simulink model "ovap_sim"  (R2025a)
settings: Solver=ode4  StartTime=0.0  StopTime=20  FixedStep=0.002  RelTol=1e-3
undefined symbols (not defined in the file): X, Y, Z
libraries: sm_lib x173, nesl_utility x72, simulink_extras x37, slpidlib x16, fl_lib x2
(part 1 of 5)
settings Model: Creator=Khang  LastModifiedBy=Khang
settings ExplorerConfigSet: InternalSimMechanicsExplorerSettings=|
  | <ExplorerConfiguration>
  | 
  |   <canonicalview>aerospace</canonicalview>
  | 
  |   <TilePanel>
  |     <TileInfo>
  |       <Tiles Columns="1" Count="1" Height="660" Rows="1" Width="1083">
  |         <Row Weight="1"/>
  |         <Column Weight="1"/>
  |         <Tile Height="1" Width="1" X="0" Y="0"/>
  |       </Tiles>
  |     </TileInfo>
  |     <SceneInfo>
  |       <SceneViewer>
  |         <IsThisViewStd>
  |           <IsStandardView>off</IsStandardView>
  |           <StandardViewName>Front</StandardViewName>
  |         </IsThisViewStd>
  |         <BGColor>
  |           <R>1</R>
  |           <G>1</G>
  |           <B>1</B>
  |           <A>1</A>
  |         </BGColor>
  |         <Camera>
  |           <DoPerspective>off</DoPerspective>
  |           <Position>
  |             <X>1.8079000547306572</X>
  |             <Y>1.5417221131491254</Y>
  |             <Z>-1.2061321654562736</Z>
  |           </Position>
  |           <Center>
  |             <X>0.0050000039551827725</X>
  |             <Y>-0.00041913422088184807</Y>
  |             <Z>-4.5055192872524335e-09</Z>
  |           </Center>
  |           <Up>
  |             <X>-0.32558894990861931</X>
  |             <Y>-0.31626154677303076</Y>
  |             <Z>-0.891050206065928</Z>
  |           </Up>
  |           <XLim>0.25728389340937141</XLim>
  |           <YLim>0.25728389340937141</YLim>
  |           <ViewLimDist>0.01</ViewLimDist>
  |         </Camera>
  |       </SceneViewer>
  |     </SceneInfo>
  |   </TilePanel>
  | 
  |   <MechEditorPanel>
  |     <GfxPanelCameraMap/>
  |     <Cameras/>
  |     <VideoCreator>
  |       <IncludeTiles>All</IncludeTiles>
  |       <IncludeTime>on</IncludeTime>
  |       <IncludeWorldFrame>off</IncludeWorldFrame>
  |       <PlaybackSpeedRatio>1</PlaybackSpeedRatio>
  |       <FrameRate>30</FrameRate>
  |       <FrameSize>auto</FrameSize>
  |       <VideoFormat>UncompressedAVI</VideoFormat>
  |     </VideoCreator>
  |   </MechEditorPanel>
  | 
  |   <PlaybackSettings>
  |     <PlaybackSpeedFactor>1</PlaybackSpeedFactor>
  |   </PlaybackSettings>
  | 
  | </ExplorerConfiguration>

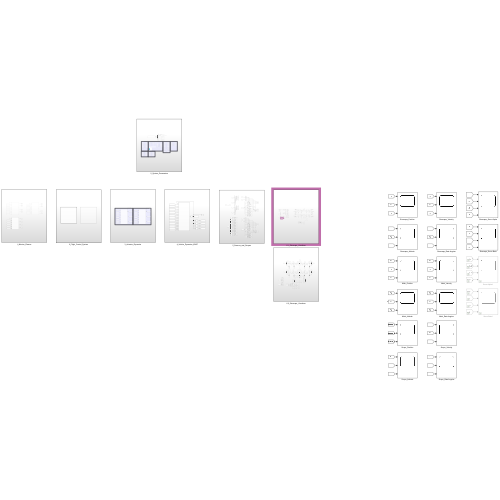
[thumbnail: Simulink's stored preview of the top-level diagram]
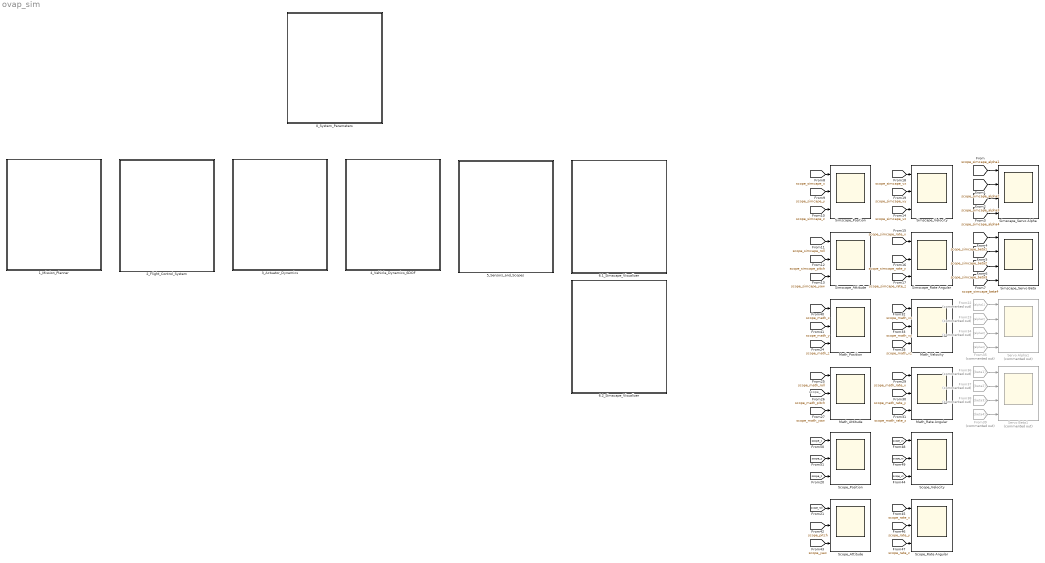
== system ovap_sim ==
  note: scope_
  0_System_Parameters : Subsystem
  1_Mission_Planner : Subsystem
  2_Flight_Control_System : Subsystem
  3_Actuator_Dynamics : Subsystem
  4_Vehicle_Dynamics_6DOF : Subsystem
  5_Sensors_and_Scopes : Subsystem
  6.1_Simscape_Visualizer : Subsystem
  6.2_Simscape_Visualizer : Subsystem
  From22 : From  Commented=on  GotoTag=alpha1
  From23 : From  Commented=on  GotoTag=alpha2
  From34 : From  Commented=on  GotoTag=alpha3
  From35 : From  Commented=on  GotoTag=alpha4
  From36 : From  Commented=on  GotoTag=beta1
  From37 : From  Commented=on  GotoTag=beta2
  From38 : From  Commented=on  GotoTag=beta3
  From39 : From  Commented=on  GotoTag=beta4
  Math_Attitude : Scope  NumInputPorts=3
      settings: ActiveDisplayYMinimum=-221.23870435466742  ActiveDisplayYMaximum=1941.5029004107885  DataLoggingVariableName=ScopeData32
  Math_Position : Scope  NumInputPorts=3
      settings: ActiveDisplayYMinimum=-1  ActiveDisplayYMaximum=1  DataLoggingVariableName=ScopeData34
  Math_Rate Angular : Scope  NumInputPorts=3
      settings: ActiveDisplayYMinimum=-1.0728968264760348E-15  ActiveDisplayYMaximum=6.562124395111157E-16  DataLoggingVariableName=ScopeData35
  Math_Velocity : Scope  NumInputPorts=3
      settings: ActiveDisplayYMinimum=-2.0436694374784938  ActiveDisplayYMaximum=7.1181854930531765  DataLoggingVariableName=ScopeData38
  Scope_Attitude : Scope  NumInputPorts=3
      settings: ActiveDisplayString=3  ActiveDisplayYMinimum=-2.4868538922904428  ActiveDisplayYMaximum=22.252327579018413  DataLoggingVariableName=ScopeData16
  Scope_Position : Scope  NumInputPorts=3
      settings: ActiveDisplayString=3  ActiveDisplayYMinimum=-1.3579834876063737  ActiveDisplayYMaximum=11.844828712328191  DataLoggingVariableName=ScopeData4
  Scope_Rate Angular : Scope  NumInputPorts=3
      settings: ActiveDisplayString=3  ActiveDisplayYMinimum=-0.388418902791342  ActiveDisplayYMaximum=0.27906120373033161  DataLoggingVariableName=ScopeData17
  Scope_Velocity : Scope  NumInputPorts=3
      settings: ActiveDisplayString=3  ActiveDisplayYMinimum=-3.4139647268091498  ActiveDisplayYMaximum=3.4772220698527239  DataLoggingVariableName=ScopeData2
  Servo Alpha1 : Scope  Commented=on  NumInputPorts=4
      settings: ActiveDisplayYMinimum=-3.9267300095298534  ActiveDisplayYMaximum=3.9256735239341554  DataLoggingVariableName=ScopeData36
  Servo Beta1 : Scope  Commented=on  NumInputPorts=4
      settings: ActiveDisplayYMinimum=-3.9267300095298534  ActiveDisplayYMaximum=3.9256735239341554  DataLoggingVariableName=ScopeData37
  Simscape_Attitude : Scope  NumInputPorts=3
      settings: ActiveDisplayYMinimum=-10.100227257036986  ActiveDisplayYMaximum=78.44868955498238
  Simscape_Position : Scope  NumInputPorts=3
      settings: ActiveDisplayYMinimum=-8.4800718375241177E-15  ActiveDisplayYMaximum=3.4315544615870859E-14
  Simscape_Rate Angular : Scope  NumInputPorts=3
      settings: ActiveDisplayYMinimum=-143.23944878270581  ActiveDisplayYMaximum=143.23944878270581  DataLoggingVariableName=ScopeData3
  Simscape_Servo Alpha : Scope  NumInputPorts=4
      settings: ActiveDisplayYMinimum=-3.9267300095298534  ActiveDisplayYMaximum=3.9256735239341554  DataLoggingVariableName=ScopeData5
  Simscape_Servo Beta : Scope  NumInputPorts=4
      settings: ActiveDisplayYMinimum=-3.9267300095298534  ActiveDisplayYMaximum=3.9256735239341554  DataLoggingVariableName=ScopeData6
  Simscape_Velocity : Scope  NumInputPorts=3
      settings: ActiveDisplayYMinimum=-143.23944878270581  ActiveDisplayYMaximum=143.23944878270581  DataLoggingVariableName=ScopeData7
  wires:
  [scope_simcape_alpha1] -> Simscape_Servo Alpha/1
  [scope_simcape_alpha2] -> Simscape_Servo Alpha/2
  [scope_simcape_alpha3] -> Simscape_Servo Alpha/3
  [scope_simcape_alpha4] -> Simscape_Servo Alpha/4
  [scope_simcape_beta1] -> Simscape_Servo Beta/1
  [scope_simcape_beta2] -> Simscape_Servo Beta/2
  [scope_simcape_beta3] -> Simscape_Servo Beta/3
  [scope_simcape_beta4] -> Simscape_Servo Beta/4
  [scope_simcape_x] -> Simscape_Position/1
  [scope_simcape_y] -> Simscape_Position/2
  [scope_simcape_z] -> Simscape_Position/3
  [scope_simcape_roll] -> Simscape_Attitude/1
  [scope_simcape_pitch] -> Simscape_Attitude/2
  [scope_simcape_yaw] -> Simscape_Attitude/3
  [scope_simcape_rate_y] -> Simscape_Rate Angular/2
  [scope_simcape_rate_z] -> Simscape_Rate Angular/3
  [scope_simcape_vy] -> Simscape_Velocity/2
  [scope_simcape_vx] -> Simscape_Velocity/1
  [scope_simcape_vz] -> Simscape_Velocity/3
  [scope_simcape_rate_x] -> Simscape_Rate Angular/1
  [scope_math_vy] -> Math_Velocity/2
  From37/1 -> Servo Beta1/2
  From34/1 -> Servo Alpha1/3
  [scope_math_y] -> Math_Position/2
  From36/1 -> Servo Beta1/1
  From22/1 -> Servo Alpha1/1
  [scope_math_pitch] -> Math_Attitude/2
  [scope_math_rate_y] -> Math_Rate Angular/2
  From38/1 -> Servo Beta1/3
  [scope_math_x] -> Math_Position/1
  [scope_math_vx] -> Math_Velocity/1
  [scope_math_roll] -> Math_Attitude/1
  [scope_math_rate_z] -> Math_Rate Angular/3
  [scope_math_vz] -> Math_Velocity/3
  From35/1 -> Servo Alpha1/4
  [scope_math_yaw] -> Math_Attitude/3
  From23/1 -> Servo Alpha1/2
  [scope_math_z] -> Math_Position/3
  [scope_math_rate_x] -> Math_Rate Angular/1
  From39/1 -> Servo Beta1/4
  [scope_rate_y] -> Scope_Rate Angular/2
  [scope_rate_z] -> Scope_Rate Angular/3
  [scope_rate_x] -> Scope_Rate Angular/1
  [scope_vy] -> Scope_Velocity/2
  [scope_yaw] -> Scope_Attitude/3
  [scope_roll] -> Scope_Attitude/1
  [scope_vz] -> Scope_Velocity/3
  [scope_vx] -> Scope_Velocity/1
  [scope_z] -> Scope_Position/3
  [scope_x] -> Scope_Position/1
  [scope_pitch] -> Scope_Attitude/2
  [scope_y] -> Scope_Position/2

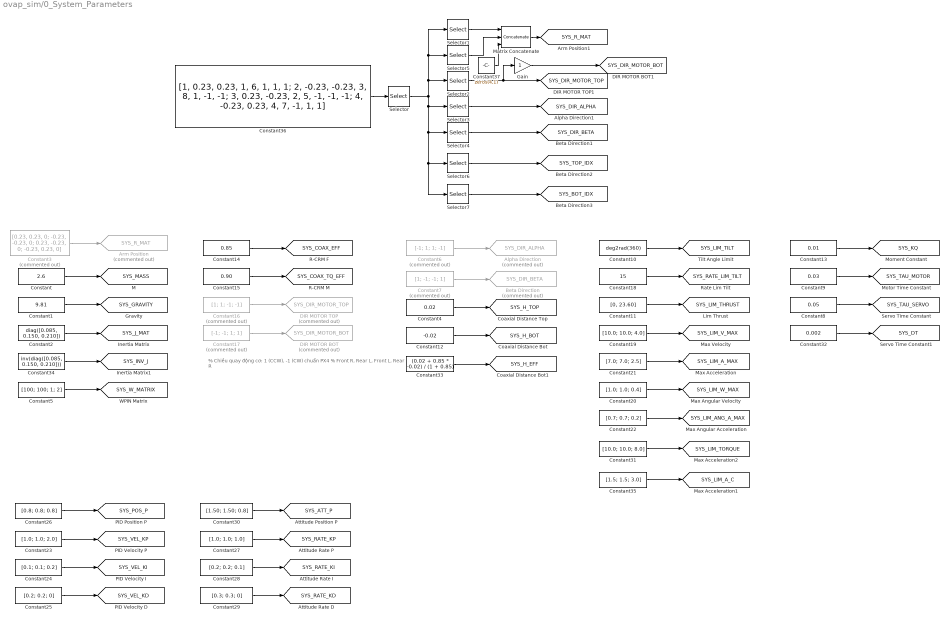
== system ovap_sim/0_System_Parameters ==
  note: % Chiều quay động cơ: 1 (CCW), -1 (CW) chuẩn PX4
      | % Front R, Rear L, Front L, Rear R
  Alpha Direction : Goto  Commented=on  GotoTag=SYS_DIR_ALPHA  TagVisibility=global
  Arm Position : Goto  Commented=on  GotoTag=SYS_R_MAT  TagVisibility=global
  Beta Direction : Goto  Commented=on  GotoTag=SYS_DIR_BETA  TagVisibility=global
  Constant : Constant  Value=2.6
  Constant1 : Constant  Value=9.81
  Constant10 : Constant  Value=deg2rad(360)
  Constant11 : Constant  Value=[0, 23.60]
  Constant12 : Constant  Value=-0.02
  Constant13 : Constant  Value=0.01
  Constant14 : Constant  Value=0.85
  Constant15 : Constant  Value=0.90
  Constant16 : Constant  Commented=on  Value=[1; 1; -1; -1]
  Constant17 : Constant  Commented=on  Value=[-1; -1; 1; 1]
  Constant18 : Constant  Value=15
  Constant19 : Constant  Value=[10.0; 10.0; 4.0]
  Constant2 : Constant  Value=diag([0.085, 0.150, 0.210])
  Constant20 : Constant  Value=[1.0; 1.0; 0.4]
  Constant21 : Constant  Value=[7.0; 7.0; 2.5]
  Constant22 : Constant  Value=[0.7; 0.7; 0.2]
  Constant23 : Constant  Value=[1.0; 1.0; 2.0]
  Constant24 : Constant  Value=[0.1; 0.1; 0.2]
  Constant25 : Constant  Value=[0.2; 0.2; 0]
  Constant26 : Constant  Value=[0.8; 0.8; 0.8]
  Constant27 : Constant  Value=[1.0; 1.0; 1.0]
  Constant28 : Constant  Value=[0.2; 0.2; 0.1]
  Constant29 : Constant  Value=[0.3; 0.3; 0]
  Constant3 : Constant  Commented=on  Value=[0.23, 0.23, 0; -0.23, -0.23, 0; 0.23, -0.23, 0; -0.23, 0.23, 0]
  Constant30 : Constant  Value=[1.50; 1.50; 0.8]
  Constant31 : Constant  Value=[10.0; 10.0; 8.0]
  Constant32 : Constant  Value=0.002
  Constant33 : Constant  Value=(0.02 + 0.85 * -0.02) / (1 + 0.85)
  Constant34 : Constant  Value=inv(diag([0.085, 0.150, 0.210]))
  Constant35 : Constant  Value=[1.5; 1.5; 3.0]
  Constant36 : Constant  Value=|
      | [1,  0.23,  0.23, 1, 6,  1,  1,  1; 
      |  2, -0.23, -0.23, 3, 8,  1, -1, -1; 
      |  3,  0.23, -0.23, 2, 5, -1, -1, -1; 
      |  4, -0.23,  0.23, 4, 7, -1,  1,  1]
  Constant37 : Constant  Value=zeros(4,1)
  Constant4 : Constant  Value=0.02
  Constant5 : Constant  Value=[100; 100; 1; 2]
  Constant6 : Constant  Commented=on  Value=[-1; 1; 1; -1]
  Constant7 : Constant  Commented=on  Value=[1; -1; -1; 1]
  Constant8 : Constant  Value=0.05
  Constant9 : Constant  Value=0.03
  DIR MOTOR BOT : Goto  Commented=on  GotoTag=SYS_DIR_MOTOR_BOT  TagVisibility=global
  DIR MOTOR TOP : Goto  Commented=on  GotoTag=SYS_DIR_MOTOR_TOP  TagVisibility=global
  Gain : Gain
  Matrix Concatenate : Concatenate  NumInputs=3  Mode=Multidimensional array  ConcatenateDimension=2
  Selector : Selector  NumberOfDimensions=2  InputPortWidth=3  IndexOptions=Select all,Index vector (dialog)  Indices=[1 3],[2 3 4 5 6 7 8]  OutputSizes=1,1
  Selector1 : Selector  NumberOfDimensions=2  InputPortWidth=3  IndexOptions=Select all,Index vector (dialog)  Indices=[1 3],1  OutputSizes=1,1
  Selector2 : Selector  NumberOfDimensions=2  InputPortWidth=3  IndexOptions=Select all,Index vector (dialog)  Indices=[1 3],5  OutputSizes=1,1
  Selector3 : Selector  NumberOfDimensions=2  InputPortWidth=3  IndexOptions=Select all,Index vector (dialog)  Indices=[1 3],6  OutputSizes=1,1
  Selector4 : Selector  NumberOfDimensions=2  InputPortWidth=3  IndexOptions=Select all,Index vector (dialog)  Indices=[1 3],7  OutputSizes=1,1
  Selector5 : Selector  NumberOfDimensions=2  InputPortWidth=3  IndexOptions=Select all,Index vector (dialog)  Indices=[1 3],2  OutputSizes=1,1
  Selector6 : Selector  NumberOfDimensions=2  InputPortWidth=3  IndexOptions=Select all,Index vector (dialog)  Indices=[1 3],3  OutputSizes=1,1
  Selector7 : Selector  NumberOfDimensions=2  InputPortWidth=3  IndexOptions=Select all,Index vector (dialog)  Indices=[1 3],4  OutputSizes=1,1
  tag scope: SYS_ATT_P=global, SYS_BOT_IDX=global, SYS_COAX_EFF=global, SYS_COAX_TQ_EFF=global, SYS_DIR_ALPHA=global, SYS_DIR_BETA=global, SYS_DIR_MOTOR_BOT=global, SYS_DIR_MOTOR_TOP=global, SYS_DT=global, SYS_GRAVITY=global, SYS_H_BOT=global, SYS_H_EFF=global, SYS_H_TOP=global, SYS_INV_J=global, SYS_J_MAT=global, SYS_KQ=global, SYS_LIM_ANG_A_MAX=global, SYS_LIM_A_C=global, SYS_LIM_A_MAX=global, SYS_LIM_THRUST=global, SYS_LIM_TILT=global, SYS_LIM_TORQUE=global, SYS_LIM_V_MAX=global, SYS_LIM_W_MAX=global, SYS_MASS=global, SYS_POS_P=global, SYS_RATE_KD=global, SYS_RATE_KI=global, SYS_RATE_KP=global, SYS_RATE_LIM_TILT=global, SYS_R_MAT=global, SYS_TAU_MOTOR=global, SYS_TAU_SERVO=global, SYS_TOP_IDX=global, SYS_VEL_KD=global, SYS_VEL_KI=global, SYS_VEL_KP=global, SYS_W_MATRIX=global
  wires:
  Constant/1 -> [SYS_MASS]
  Constant1/1 -> [SYS_GRAVITY]
  Constant2/1 -> [SYS_J_MAT]
  Constant3/1 -> Arm Position/1
  Constant5/1 -> [SYS_W_MATRIX]
  Constant6/1 -> Alpha Direction/1
  Constant7/1 -> Beta Direction/1
  Constant9/1 -> [SYS_TAU_MOTOR]
  Constant8/1 -> [SYS_TAU_SERVO]
  Constant10/1 -> [SYS_LIM_TILT]
  Constant11/1 -> [SYS_LIM_THRUST]
  Constant4/1 -> [SYS_H_TOP]
  Constant12/1 -> [SYS_H_BOT]
  Constant13/1 -> [SYS_KQ]
  Constant14/1 -> [SYS_COAX_EFF]
  Constant15/1 -> [SYS_COAX_TQ_EFF]
  Constant17/1 -> DIR MOTOR BOT/1
  Constant16/1 -> DIR MOTOR TOP/1
  Constant18/1 -> [SYS_RATE_LIM_TILT]
  Constant21/1 -> [SYS_LIM_A_MAX]
  Constant20/1 -> [SYS_LIM_W_MAX]
  Constant19/1 -> [SYS_LIM_V_MAX]
  Constant22/1 -> [SYS_LIM_ANG_A_MAX]
  Constant23/1 -> [SYS_VEL_KP]
  Constant24/1 -> [SYS_VEL_KI]
  Constant26/1 -> [SYS_POS_P]
  Constant25/1 -> [SYS_VEL_KD]
  Constant28/1 -> [SYS_RATE_KI]
  Constant29/1 -> [SYS_RATE_KD]
  Constant30/1 -> [SYS_ATT_P]
  Constant27/1 -> [SYS_RATE_KP]
  Constant31/1 -> [SYS_LIM_TORQUE]
  Constant32/1 -> [SYS_DT]
  Constant33/1 -> [SYS_H_EFF]
  Constant34/1 -> [SYS_INV_J]
  Constant35/1 -> [SYS_LIM_A_C]
  Constant36/1 -> Selector/1
  Selector/1 -> Selector7/1, Selector6/1, Selector4/1, Selector3/1, Selector2/1, Selector1/1, Selector5/1
  Selector2/1 -> Gain/1, [SYS_DIR_MOTOR_TOP]
  Selector3/1 -> [SYS_DIR_ALPHA]
  Selector4/1 -> [SYS_DIR_BETA]
  Constant37/1 -> Matrix Concatenate/3
  Selector1/1 -> Matrix Concatenate/1
  Matrix Concatenate/1 -> [SYS_R_MAT]
  Selector5/1 -> Matrix Concatenate/2
  Selector6/1 -> [SYS_TOP_IDX]
  Selector7/1 -> [SYS_BOT_IDX]
  Gain/1 -> [SYS_DIR_MOTOR_BOT]

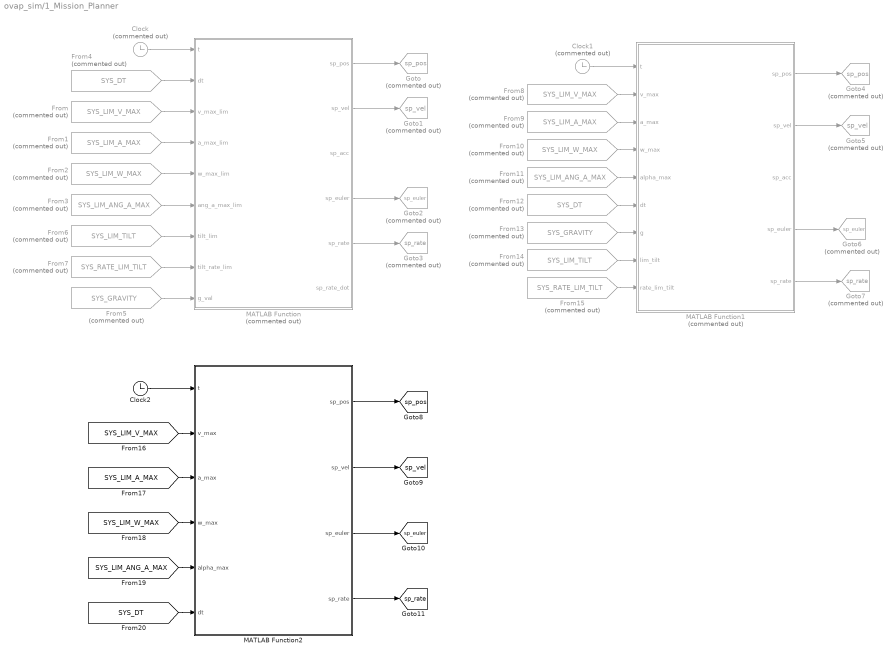
== system ovap_sim/1_Mission_Planner ==
  Clock : Clock  Commented=on
  Clock1 : Clock  Commented=on
  Clock2 : Clock
  From : From  Commented=on  GotoTag=SYS_LIM_V_MAX  TagVisibility=global
  From1 : From  Commented=on  GotoTag=SYS_LIM_A_MAX  TagVisibility=global
  From10 : From  Commented=on  GotoTag=SYS_LIM_W_MAX  TagVisibility=global
  From11 : From  Commented=on  GotoTag=SYS_LIM_ANG_A_MAX  TagVisibility=global
  From12 : From  Commented=on  GotoTag=SYS_DT  TagVisibility=global
  From13 : From  Commented=on  GotoTag=SYS_GRAVITY  TagVisibility=global
  From14 : From  Commented=on  GotoTag=SYS_LIM_TILT  TagVisibility=global
  From15 : From  Commented=on  GotoTag=SYS_RATE_LIM_TILT  TagVisibility=global
  From2 : From  Commented=on  GotoTag=SYS_LIM_W_MAX  TagVisibility=global
  From3 : From  Commented=on  GotoTag=SYS_LIM_ANG_A_MAX  TagVisibility=global
  From4 : From  Commented=on  GotoTag=SYS_DT  TagVisibility=global
  From5 : From  Commented=on  GotoTag=SYS_GRAVITY  TagVisibility=global
  From6 : From  Commented=on  GotoTag=SYS_LIM_TILT  TagVisibility=global
  From7 : From  Commented=on  GotoTag=SYS_RATE_LIM_TILT  TagVisibility=global
  From8 : From  Commented=on  GotoTag=SYS_LIM_V_MAX  TagVisibility=global
  From9 : From  Commented=on  GotoTag=SYS_LIM_A_MAX  TagVisibility=global
  Goto : Goto  Commented=on  GotoTag=sp_pos  TagVisibility=global
  Goto1 : Goto  Commented=on  GotoTag=sp_vel  TagVisibility=global
  Goto2 : Goto  Commented=on  GotoTag=sp_euler  TagVisibility=global
  Goto3 : Goto  Commented=on  GotoTag=sp_rate  TagVisibility=global
  Goto4 : Goto  Commented=on  GotoTag=sp_pos  TagVisibility=global
  Goto5 : Goto  Commented=on  GotoTag=sp_vel  TagVisibility=global
  Goto6 : Goto  Commented=on  GotoTag=sp_euler  TagVisibility=global
  Goto7 : Goto  Commented=on  GotoTag=sp_rate  TagVisibility=global
  MATLAB Function : MATLAB Function  Commented=on  TreatAsAtomicUnit=on
  MATLAB Function1 : MATLAB Function  Commented=on  TreatAsAtomicUnit=on
  MATLAB Function2 : MATLAB Function  TreatAsAtomicUnit=on
  tag scope: sp_euler=global, sp_pos=global, sp_rate=global, sp_vel=global
  wires:
  MATLAB Function/1(sp_pos) -> Goto/1
  MATLAB Function/5(sp_rate) -> Goto3/1
  MATLAB Function/2(sp_vel) -> Goto1/1
  MATLAB Function/4(sp_euler) -> Goto2/1
  From15/1 -> MATLAB Function1/9(rate_lim_tilt)
  From11/1 -> MATLAB Function1/5(alpha_max)
  From13/1 -> MATLAB Function1/7(g)
  MATLAB Function1/5(sp_rate) -> Goto7/1
  From9/1 -> MATLAB Function1/3(a_max)
  From12/1 -> MATLAB Function1/6(dt)
  From14/1 -> MATLAB Function1/8(lim_tilt)
  Clock1/1 -> MATLAB Function1/1(t)
  MATLAB Function1/2(sp_vel) -> Goto5/1
  From10/1 -> MATLAB Function1/4(w_max)
  MATLAB Function1/1(sp_pos) -> Goto4/1
  MATLAB Function1/4(sp_euler) -> Goto6/1
  From8/1 -> MATLAB Function1/2(v_max)
  Clock/1 -> MATLAB Function/1(t)
  From4/1 -> MATLAB Function/2(dt)
  From/1 -> MATLAB Function/3(v_max_lim)
  From1/1 -> MATLAB Function/4(a_max_lim)
  From2/1 -> MATLAB Function/5(w_max_lim)
  From3/1 -> MATLAB Function/6(ang_a_max_lim)
  From6/1 -> MATLAB Function/7(tilt_lim)
  From7/1 -> MATLAB Function/8(tilt_rate_lim)
  From5/1 -> MATLAB Function/9(g_val)
  MATLAB Function2/3(sp_euler) -> [sp_euler]
  [SYS_LIM_W_MAX] -> MATLAB Function2/4(w_max)
  [SYS_DT] -> MATLAB Function2/6(dt)
  Clock2/1 -> MATLAB Function2/1(t)
  [SYS_LIM_V_MAX] -> MATLAB Function2/2(v_max)
  [SYS_LIM_A_MAX] -> MATLAB Function2/3(a_max)
  [SYS_LIM_ANG_A_MAX] -> MATLAB Function2/5(alpha_max)
  MATLAB Function2/2(sp_vel) -> [sp_vel]
  MATLAB Function2/4(sp_rate) -> [sp_rate]
  MATLAB Function2/1(sp_pos) -> [sp_pos]

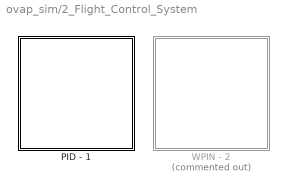
== system ovap_sim/2_Flight_Control_System ==
  PID - 1 : Subsystem
  WPIN - 2 : Subsystem  Commented=on

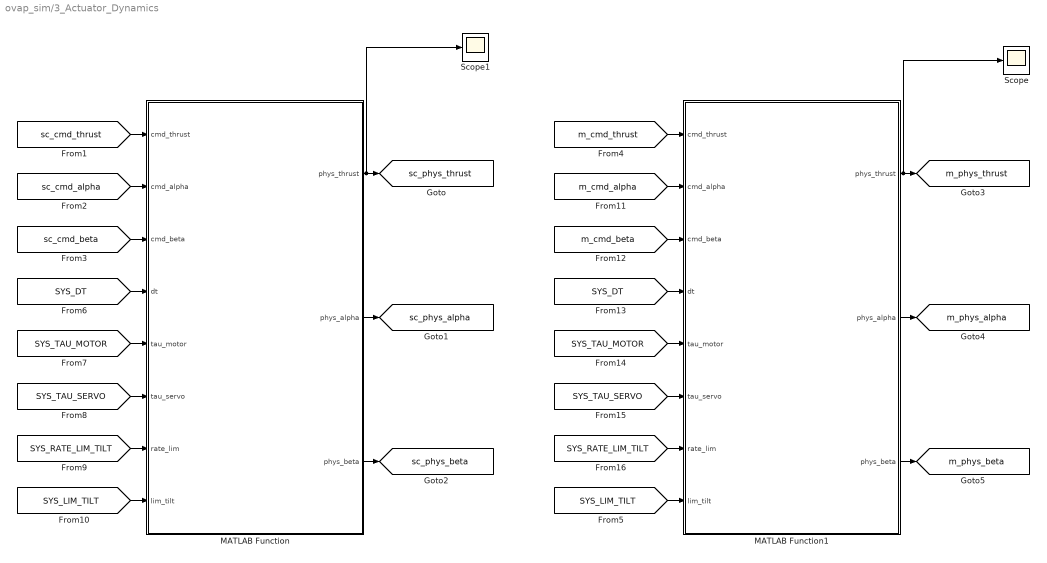
== system ovap_sim/3_Actuator_Dynamics ==
  MATLAB Function : MATLAB Function  TreatAsAtomicUnit=on
  MATLAB Function1 : MATLAB Function  TreatAsAtomicUnit=on
  Scope : Scope
      settings: ActiveDisplayYMinimum=-0.43208562670916689  ActiveDisplayYMaximum=5.9390843457396461  DataLoggingVariableName=ScopeData26
  Scope1 : Scope
      settings: ActiveDisplayYMinimum=-0.34916650190561566  ActiveDisplayYMaximum=5.1928122225076851  DataLoggingVariableName=ScopeData27
  tag scope: m_phys_alpha=global, m_phys_beta=global, m_phys_thrust=global, sc_phys_alpha=global, sc_phys_beta=global, sc_phys_thrust=global
  wires:
  [SYS_DT] -> MATLAB Function/4(dt)
  [SYS_TAU_MOTOR] -> MATLAB Function/5(tau_motor)
  [SYS_TAU_SERVO] -> MATLAB Function/6(tau_servo)
  [SYS_RATE_LIM_TILT] -> MATLAB Function/7(rate_lim)
  [SYS_LIM_TILT] -> MATLAB Function/8(lim_tilt)
  MATLAB Function/1(phys_thrust) -> Scope1/1, [sc_phys_thrust]
  MATLAB Function/2(phys_alpha) -> [sc_phys_alpha]
  MATLAB Function/3(phys_beta) -> [sc_phys_beta]
  [sc_cmd_thrust] -> MATLAB Function/1(cmd_thrust)
  [sc_cmd_alpha] -> MATLAB Function/2(cmd_alpha)
  [sc_cmd_beta] -> MATLAB Function/3(cmd_beta)
  MATLAB Function1/1(phys_thrust) -> Scope/1, [m_phys_thrust]
  [SYS_TAU_MOTOR] -> MATLAB Function1/5(tau_motor)
  [m_cmd_beta] -> MATLAB Function1/3(cmd_beta)
  [SYS_DT] -> MATLAB Function1/4(dt)
  [SYS_LIM_TILT] -> MATLAB Function1/8(lim_tilt)
  MATLAB Function1/3(phys_beta) -> [m_phys_beta]
  MATLAB Function1/2(phys_alpha) -> [m_phys_alpha]
  [m_cmd_alpha] -> MATLAB Function1/2(cmd_alpha)
  [SYS_RATE_LIM_TILT] -> MATLAB Function1/7(rate_lim)
  [m_cmd_thrust] -> MATLAB Function1/1(cmd_thrust)
  [SYS_TAU_SERVO] -> MATLAB Function1/6(tau_servo)

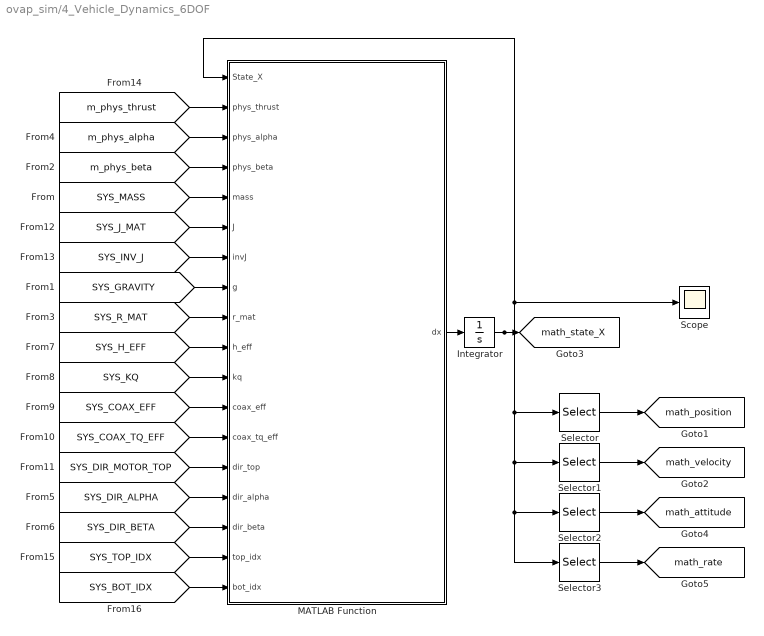
== system ovap_sim/4_Vehicle_Dynamics_6DOF ==
  Integrator : Integrator  InitialCondition=zeros(12,1)
  MATLAB Function : MATLAB Function  TreatAsAtomicUnit=on
  Scope : Scope
      settings: ActiveDisplayYMinimum=-6.3018139743557592E-12  ActiveDisplayYMaximum=5.6560338694093331E-11  DataLoggingVariableName=ScopeData19
  Selector : Selector  InputPortWidth=12  IndexOptions=Index vector (dialog)  Indices=[1:3]  OutputSizes=1
  Selector1 : Selector  InputPortWidth=12  IndexOptions=Index vector (dialog)  Indices=[4:6]  OutputSizes=1
  Selector2 : Selector  InputPortWidth=12  IndexOptions=Index vector (dialog)  Indices=[7:9]  OutputSizes=1
  Selector3 : Selector  InputPortWidth=12  IndexOptions=Index vector (dialog)  Indices=[10:12]  OutputSizes=1
  tag scope: math_attitude=global, math_position=global, math_rate=global, math_state_X=global, math_velocity=global
  wires:
  MATLAB Function/1(dx) -> Integrator/1
  [SYS_MASS] -> MATLAB Function/5(mass)
  [SYS_GRAVITY] -> MATLAB Function/8(g)
  [SYS_DIR_ALPHA] -> MATLAB Function/15(dir_alpha)
  [SYS_DIR_BETA] -> MATLAB Function/16(dir_beta)
  Integrator/1 -> Selector3/1, Selector2/1, Selector1/1, Selector/1, Scope/1, MATLAB Function/1(State_X), [math_state_X]
  [SYS_H_EFF] -> MATLAB Function/10(h_eff)
  [SYS_COAX_EFF] -> MATLAB Function/12(coax_eff)
  [SYS_COAX_TQ_EFF] -> MATLAB Function/13(coax_tq_eff)
  [SYS_DIR_MOTOR_TOP] -> MATLAB Function/14(dir_top)
  [SYS_KQ] -> MATLAB Function/11(kq)
  [SYS_J_MAT] -> MATLAB Function/6(J)
  [SYS_INV_J] -> MATLAB Function/7(invJ)
  [SYS_R_MAT] -> MATLAB Function/9(r_mat)
  [m_phys_thrust] -> MATLAB Function/2(phys_thrust)
  [m_phys_alpha] -> MATLAB Function/3(phys_alpha)
  [m_phys_beta] -> MATLAB Function/4(phys_beta)
  Selector/1 -> [math_position]
  Selector3/1 -> [math_rate]
  Selector1/1 -> [math_velocity]
  [SYS_TOP_IDX] -> MATLAB Function/17(top_idx)
  [SYS_BOT_IDX] -> MATLAB Function/18(bot_idx)
  Selector2/1 -> [math_attitude]

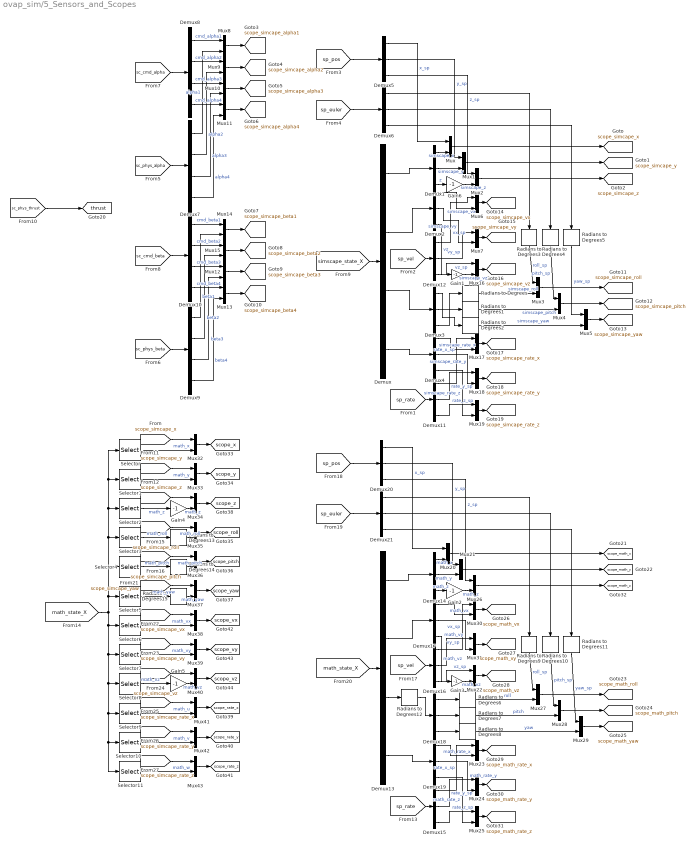
== system ovap_sim/5_Sensors_and_Scopes ==
  Demux{,7..10,13} (6 alike) : Demux
  Demux{1..6,11..12,14..21} (16 alike) : Demux  Outputs=3
  Gain{1..6} (6 alike) : Gain  Gain=-1
  Mux{,1..43} (44 alike) : Mux  Inputs=2
  Radians to Degrees{,1..15} (16 alike) : simulink_extras/Transformations/Radians to Degrees
  Selector : Selector  InputPortWidth=12  IndexOptions=Index vector (dialog)  Indices=1  OutputSizes=1
  Selector1 : Selector  InputPortWidth=12  IndexOptions=Index vector (dialog)  Indices=2  OutputSizes=1
  Selector10 : Selector  InputPortWidth=12  IndexOptions=Index vector (dialog)  Indices=11  OutputSizes=1
  Selector11 : Selector  InputPortWidth=12  IndexOptions=Index vector (dialog)  Indices=12  OutputSizes=1
  Selector2 : Selector  InputPortWidth=12  IndexOptions=Index vector (dialog)  Indices=3  OutputSizes=1
  Selector3 : Selector  InputPortWidth=12  IndexOptions=Index vector (dialog)  Indices=7  OutputSizes=1
  Selector4 : Selector  InputPortWidth=12  IndexOptions=Index vector (dialog)  Indices=8  OutputSizes=1
  Selector5 : Selector  InputPortWidth=12  IndexOptions=Index vector (dialog)  Indices=9  OutputSizes=1
  Selector6 : Selector  InputPortWidth=12  IndexOptions=Index vector (dialog)  Indices=4  OutputSizes=1
  Selector7 : Selector  InputPortWidth=12  IndexOptions=Index vector (dialog)  Indices=5  OutputSizes=1
  Selector8 : Selector  InputPortWidth=12  IndexOptions=Index vector (dialog)  Indices=6  OutputSizes=1
  Selector9 : Selector  InputPortWidth=12  IndexOptions=Index vector (dialog)  Indices=10  OutputSizes=1
  tag scope: scope_math_pitch=global, scope_math_rate_x=global, scope_math_rate_y=global, scope_math_rate_z=global, scope_math_roll=global, scope_math_vx=global, scope_math_vy=global, scope_math_vz=global, scope_math_x=global, scope_math_y=global, scope_math_yaw=global, scope_math_z=global, scope_pitch=global, scope_rate_x=global, scope_rate_y=global, scope_rate_z=global, scope_roll=global, scope_simcape_alpha1=global, scope_simcape_alpha2=global, scope_simcape_alpha3=global, scope_simcape_alpha4=global, scope_simcape_beta1=global, scope_simcape_beta2=global, scope_simcape_beta3=global, scope_simcape_beta4=global, scope_simcape_pitch=global, scope_simcape_rate_x=global, scope_simcape_rate_y=global, scope_simcape_rate_z=global, scope_simcape_roll=global, scope_simcape_vx=global, scope_simcape_vy=global, scope_simcape_vz=global, scope_simcape_x=global, scope_simcape_y=global, scope_simcape_yaw=global, scope_simcape_z=global, scope_vx=global, scope_vy=global, scope_vz=global, scope_x=global, scope_y=global, scope_yaw=global, scope_z=global, thrust=global
  wires:
  [simscape_state_X] -> Demux/1
  Demux/1 -> Demux1/1
  Demux/2 -> Demux2/1
  Demux/4 -> Demux4/1
  Demux/3 -> Demux3/1
  [sp_pos] -> Demux5/1
  Demux5/1 -> Mux/1  "x_sp"
  Demux1/1 -> Mux/2  "simscape_x"
  Mux/1 -> [scope_simcape_x]
  Demux5/2 -> Mux1/1  "y_sp"
  Demux5/3 -> Mux2/1  "z_sp"
  Demux1/2 -> Mux1/2  "simscape_y"
  Demux1/3 -> Gain6/1  "z"
  Mux1/1 -> [scope_simcape_y]
  Mux2/1 -> [scope_simcape_z]
  [sp_euler] -> Demux6/1
  Demux2/1 -> Mux6/2  "simscape_vx"
  Demux2/2 -> Mux7/2  "simscape_vy"
  [sc_cmd_alpha] -> Demux8/1
  Demux8/1 -> Mux8/1  "cmd_alpha1"
  Demux7/1 -> Mux8/2  "alpha1"
  Demux8/2 -> Mux9/1  "cmd_alpha2"
  Demux7/2 -> Mux9/2  "alpha2"
  Demux8/3 -> Mux10/1  "cmd_alpha3"
  Demux7/3 -> Mux10/2  "alpha3"
  Demux8/4 -> Mux11/1  "cmd_alpha4"
  Demux7/4 -> Mux11/2  "alpha4"
  Demux10/3 -> Mux12/1  "cmd_beta3"
  Demux9/2 -> Mux15/2  "beta2"
  Demux10/2 -> Mux15/1  "cmd_beta2"
  Demux10/1 -> Mux14/1  "cmd_beta1"
  Demux9/3 -> Mux12/2  "beta3"
  Demux10/4 -> Mux13/1  "cmd_beta4"
  Demux9/1 -> Mux14/2  "beta1"
  Demux9/4 -> Mux13/2  "beta4"
  [sc_cmd_beta] -> Demux10/1
  [sc_phys_beta] -> Demux9/1
  Mux8/1 -> [scope_simcape_alpha1]
  Mux9/1 -> [scope_simcape_alpha2]
  Mux10/1 -> [scope_simcape_alpha3]
  Mux11/1 -> [scope_simcape_alpha4]
  Mux15/1 -> [scope_simcape_beta2]
  Mux12/1 -> [scope_simcape_beta3]
  Mux13/1 -> [scope_simcape_beta4]
  Mux14/1 -> [scope_simcape_beta1]
  Mux3/1 -> [scope_simcape_roll]
  Mux4/1 -> [scope_simcape_pitch]
  Mux5/1 -> [scope_simcape_yaw]
  Radians to Degrees/1 -> Mux3/2  "simscape_roll"
  Radians to Degrees1/1 -> Mux4/2  "simscape_pitch"
  Radians to Degrees3/1 -> Mux3/1  "roll_sp"
  Radians to Degrees4/1 -> Mux4/1  "pitch_sp"
  Radians to Degrees5/1 -> Mux5/1  "yaw_sp"
  [sp_rate] -> Demux11/1
  [sp_vel] -> Demux12/1
  Demux12/1 -> Mux6/1  "vx_sp"
  Demux12/2 -> Mux7/1  "vy_sp"
  Demux12/3 -> Mux16/1  "vz_sp"
  Mux6/1 -> [scope_simcape_vx]
  Mux7/1 -> [scope_simcape_vy]
  Mux16/1 -> [scope_simcape_vz]
  Mux19/1 -> [scope_simcape_rate_z]
  Demux11/3 -> Mux19/1  "rate_z_sp"
  Demux4/1 -> Mux17/2  "simscape_rate_x"
  Demux11/2 -> Mux18/1  "rate_y_sp"
  Demux4/2 -> Mux18/2  "simscape_rate_y"
  Mux18/1 -> [scope_simcape_rate_y]
  Demux4/3 -> Mux19/2  "simscape_rate_z"
  Mux17/1 -> [scope_simcape_rate_x]
  Demux11/1 -> Mux17/1  "rate_x_sp"
  [sc_phys_thrust] -> [thrust]
  [sc_phys_alpha] -> Demux7/1
  Gain6/1 -> Mux2/2  "simscape_z"
  Radians to Degrees2/1 -> Mux5/2  "simscape_yaw"
  Demux3/1 -> Radians to Degrees2/1
  Demux3/2 -> Radians to Degrees1/1
  Demux3/3 -> Radians to Degrees/1
  Demux6/1 -> Radians to Degrees3/1
  Demux6/3 -> Radians to Degrees5/1
  Demux6/2 -> Radians to Degrees4/1
  Demux17/2 -> Mux31/2  "math_vy"
  Demux21/1 -> Radians to Degrees9/1
  Demux13/2 -> Demux17/1
  Mux22/1 -> [scope_math_vz]
  Mux28/1 -> [scope_math_pitch]
  Mux30/1 -> [scope_math_vx]
  [sp_rate] -> Demux15/1
  [math_state_X] -> Demux13/1
  Mux26/1 -> [scope_math_z]
  Demux15/1 -> Mux23/1  "rate_x_sp"
  Demux16/3 -> Mux22/1  "vz_sp"
  Demux17/1 -> Mux30/2  "math_vx"
  Demux15/3 -> Mux25/1  "rate_z_sp"
  Mux29/1 -> [scope_math_yaw]
  Demux19/2 -> Mux24/2  "math_rate_y"
  Mux24/1 -> [scope_math_rate_y]
  Mux23/1 -> [scope_math_rate_x]
  Demux19/3 -> Mux25/2  "math_rate_z"
  Mux21/1 -> [scope_math_y]
  Mux25/1 -> [scope_math_rate_z]
  [sp_vel] -> Demux16/1
  Demux18/2 -> Radians to Degrees7/1
  Demux19/1 -> Mux23/2  "math_rate_x"
  Demux14/1 -> Mux20/2  "math_x"
  Radians to Degrees8/1 -> Mux29/2  "yaw"
  Radians to Degrees9/1 -> Mux27/1  "roll_sp"
  [sp_euler] -> Demux21/1
  Radians to Degrees11/1 -> Mux29/1  "yaw_sp"
  Radians to Degrees10/1 -> Mux28/1  "pitch_sp"
  Demux14/3 -> Gain2/1  "math_z"
  Demux21/2 -> Radians to Degrees10/1
  Demux21/3 -> Radians to Degrees11/1
  Demux13/1 -> Demux14/1
  Mux31/1 -> [scope_math_vy]
  Demux16/2 -> Mux31/1  "vy_sp"
  Demux16/1 -> Mux30/1  "vx_sp"
  [sp_pos] -> Demux20/1
  Demux20/2 -> Mux21/1  "y_sp"
  Demux15/2 -> Mux24/1  "rate_y_sp"
  Demux14/2 -> Mux21/2  "math_y"
  Mux20/1 -> [scope_math_x]
  Radians to Degrees7/1 -> Mux28/2  "pitch"
  Radians to Degrees6/1 -> Mux27/2  "roll"
  Demux13/4 -> Demux19/1
  Demux20/1 -> Mux20/1  "x_sp"
  Mux27/1 -> [scope_math_roll]
  Demux20/3 -> Mux26/1  "z_sp"
  Mux32/1 -> [scope_x]
  Mux33/1 -> [scope_y]
  Mux34/1 -> [scope_z]
  [scope_simcape_z] -> Mux34/1
  [scope_simcape_y] -> Mux33/1
  [scope_simcape_x] -> Mux32/1
  Selector/1 -> Mux32/2  "math_x"
  Selector1/1 -> Mux33/2  "math_y"
  Selector2/1 -> Gain4/1  "math_z"
  Selector5/1 -> Radians to Degrees15/1  "math_yaw"
  [scope_simcape_roll] -> Mux35/1
  Mux35/1 -> [scope_roll]
  [scope_simcape_pitch] -> Mux36/1
  Selector4/1 -> Radians to Degrees14/1  "math_pitch"
  Mux36/1 -> [scope_pitch]
  [scope_simcape_yaw] -> Mux37/1
  Selector3/1 -> Radians to Degrees13/1  "math_roll"
  Mux37/1 -> [scope_yaw]
  [scope_simcape_rate_x] -> Mux41/1
  [scope_simcape_vx] -> Mux38/1
  [scope_simcape_vy] -> Mux39/1
  [scope_simcape_rate_z] -> Mux43/1
  Selector10/1 -> Mux42/2  "math_v"
  Selector8/1 -> Gain5/1  "math_vz"
  Selector11/1 -> Mux43/2  "math_w"
  Selector9/1 -> Mux41/2  "math_u"
  Mux38/1 -> [scope_vx]
  Mux42/1 -> [scope_rate_y]
  Selector7/1 -> Mux39/2  "math_vy"
  Mux41/1 -> [scope_rate_x]
  Mux39/1 -> [scope_vy]
  [scope_simcape_vz] -> Mux40/1
  Mux43/1 -> [scope_rate_z]
  Selector6/1 -> Mux38/2  "math_vx"
  Mux40/1 -> [scope_vz]
  [scope_simcape_rate_y] -> Mux42/1
  [math_state_X] -> Selector11/1, Selector10/1, Selector9/1, Selector8/1, Selector7/1, Selector6/1, Selector2/1, Selector1/1, Selector/1, Selector3/1, Selector4/1, Selector5/1
  Gain1/1 -> Mux16/2  "simscape_vz"
  Demux2/3 -> Gain1/1  "vz"
  Gain2/1 -> Mux26/2  "math_z"
  Demux18/1 -> Radians to Degrees6/1
  Demux18/3 -> Radians to Degrees8/1
  Demux17/3 -> Gain3/1  "math_vz"
  Gain3/1 -> Mux22/2  "math_vz"
  Gain4/1 -> Mux34/2  "math_z"
  Gain5/1 -> Mux40/2  "math_vz"
  Demux13/3 -> Radians to Degrees12/1
  Radians to Degrees12/1 -> Demux18/1
  Radians to Degrees13/1 -> Mux35/2  "math_roll"
  Radians to Degrees14/1 -> Mux36/2  "math_pitch"
  Radians to Degrees15/1 -> Mux37/2  "math_yaw"
